simulink model "ThreePhasePFC_threePhase"  (R2018a)
settings: Solver=VariableStepAuto  StartTime=0.0  StopTime=0.6  RelTol=1e-3  AbsTol=1e-3  EnableMultiTasking=on
undefined symbols (not defined in the file or in its folder): Gain, L_Reactor, R_Reactor, Vac, Vdc, Vdc_offset
libraries: powerlib x36, powerlib_meascontrol x3
settings Model: Creator=snow_  LastModifiedBy=snow_
settings SolverCC: AutoScaleAbsTol=off
settings DataIOCC: LimitDataPoints=on  MaxDataPoints=10000
settings OptimizationCC: LifeSpan=inf
settings DebuggingCC: AllowSymbolicDim=off  SFUnexpectedBacktrackingDiag=warning  SFNoUnconditionalDefaultTransitionDiag=warning  SFExecutionAtInitializationDiag=none
settings CodeAppCC: StateflowObjectComments=on
settings GRTTargetCC: TargetLangStandard=C89/C90 (ANSI)  GeneratePreprocessorConditionals=Disable all
settings ConfigComp: CovMetricSettings=dw  CovHtmlReporting=on  CovSaveCumulativeToWorkspaceVar=on  CovSaveSingleToWorkspaceVar=on  CovExternalEMLEnable=off  CovSFcnEnable=off
settings SimscapeCC: SimscapeLogType=all  SimscapeLogDataHistory=10000

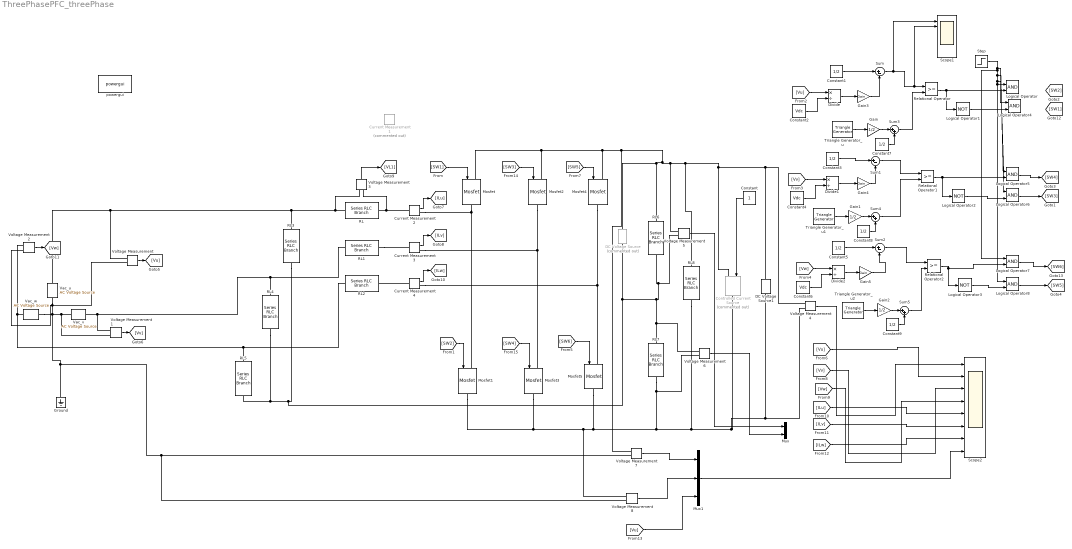
== system ThreePhasePFC_threePhase ==
  Constant : Constant
  Constant{1,3,5,7..9} (6 alike) : Constant  Value=1/2
  Constant2 : Constant  Value=Vdc
  Constant4 : Constant  Value=Vdc
  Constant6 : Constant  Value=Vdc
  Controlled Current Source : powerlib/Electrical Sources/Controlled Current Source  Commented=on  Initialize=on  Source_Type=AC  Amplitude=0  Phase=0  Frequency=0  Measurements=None
  Current Measurement1 : powerlib/Measurements/Current Measurement  Commented=on  PhasorSimulation=off  OutputType=Complex  PSBequivalent=0
  Current Measurement2 : powerlib/Measurements/Current Measurement  PhasorSimulation=off  OutputType=Complex  PSBequivalent=0
  Current Measurement3 : powerlib/Measurements/Current Measurement  PhasorSimulation=off  OutputType=Complex  PSBequivalent=0
  Current Measurement4 : powerlib/Measurements/Current Measurement  PhasorSimulation=off  OutputType=Complex  PSBequivalent=0
  DC Voltage Source : powerlib/Electrical Sources/DC Voltage Source  Commented=on  Amplitude=Vdc_offset  Measurements=None
  DC Voltage Source1 : powerlib/Electrical Sources/DC Voltage Source  Amplitude=Vdc  Measurements=None
  Divide : Product  Inputs=*/
  Divide1 : Product  Inputs=*/
  Divide2 : Product  Inputs=*/
  Gain : Gain  Gain=1/2
  Gain1 : Gain  Gain=1/2
  Gain2 : Gain  Gain=1/2
  Gain3 : Gain  Gain=Gain
  Gain4 : Gain  Gain=Gain
  Gain5 : Gain  Gain=Gain
  Ground : powerlib/Elements/Ground  LConnTagsString=a
  Logical Operator{,4..8} (6 alike) : Logic  AllPortsSameDT=off  OutDataTypeStr=boolean
  Logical Operator1 : Logic  Operator=NOT  AllPortsSameDT=off  OutDataTypeStr=boolean
  Logical Operator2 : Logic  Operator=NOT  AllPortsSameDT=off  OutDataTypeStr=boolean
  Logical Operator3 : Logic  Operator=NOT  AllPortsSameDT=off  OutDataTypeStr=boolean
  Mosfet{,1..5} (6 alike) : powerlib/Power Electronics/Mosfet  Ron=0.01  Lon=0  Rd=0.01  Vfd=0.7  IC=0  Rs=1e5  Cs=inf  Measurements=off
  Mux : Mux  Inputs=2
  Mux1 : Mux  Inputs=3
  RL : powerlib/Elements/Series RLC Branch  LConnTagsString=__new0  RConnTagsString=__new0  BranchType=RL  Resistance=R_Reactor  Inductance=L_Reactor  SetiL0=off  InitialCurrent=0  Capacitance=1e-6  Setx0=off  InitialVoltage=0  Measurements=None
      settings: AttributesFormatString=|
      | L=%<Inductance> H
      | R=%<Resistance> Ohm
  RL1 : powerlib/Elements/Series RLC Branch  LConnTagsString=__new0  RConnTagsString=__new0  BranchType=RL  Resistance=R_Reactor  Inductance=L_Reactor  SetiL0=off  InitialCurrent=0  Capacitance=1e-6  Setx0=off  InitialVoltage=0  Measurements=None
      settings: AttributesFormatString=|
      | L=%<Inductance> H
      | R=%<Resistance> Ohm
  RL2 : powerlib/Elements/Series RLC Branch  LConnTagsString=__new0  RConnTagsString=__new0  BranchType=RL  Resistance=R_Reactor  Inductance=L_Reactor  SetiL0=off  InitialCurrent=0  Capacitance=1e-6  Setx0=off  InitialVoltage=0  Measurements=None
      settings: AttributesFormatString=|
      | L=%<Inductance> H
      | R=%<Resistance> Ohm
  RL3 : powerlib/Elements/Series RLC Branch  LConnTagsString=__new0  RConnTagsString=__new0  BranchType=RC  Resistance=R_Reactor  Inductance=L_Reactor  SetiL0=off  InitialCurrent=0  Capacitance=20e-6  Setx0=off  InitialVoltage=0  Measurements=None
      settings: AttributesFormatString=C=%<Capacitance>F
  RL4 : powerlib/Elements/Series RLC Branch  LConnTagsString=__new0  RConnTagsString=__new0  BranchType=RC  Resistance=R_Reactor  Inductance=L_Reactor  SetiL0=off  InitialCurrent=0  Capacitance=20e-6  Setx0=off  InitialVoltage=0  Measurements=None
      settings: AttributesFormatString=C=%<Capacitance>F
  RL5 : powerlib/Elements/Series RLC Branch  LConnTagsString=__new0  RConnTagsString=__new0  BranchType=RC  Resistance=R_Reactor  Inductance=L_Reactor  SetiL0=off  InitialCurrent=0  Capacitance=20e-6  Setx0=off  InitialVoltage=0  Measurements=None
      settings: AttributesFormatString=C=%<Capacitance>F
  RL6 : powerlib/Elements/Series RLC Branch  LConnTagsString=__new0  RConnTagsString=__new0  BranchType=RC  Resistance=R_Reactor  Inductance=L_Reactor  SetiL0=off  InitialCurrent=0  Capacitance=20e-6  Setx0=on  InitialVoltage=Vdc/2  Measurements=None
      settings: AttributesFormatString=C=%<Capacitance>F
  RL7 : powerlib/Elements/Series RLC Branch  LConnTagsString=__new0  RConnTagsString=__new0  BranchType=RC  Resistance=R_Reactor  Inductance=L_Reactor  SetiL0=off  InitialCurrent=0  Capacitance=20e-6  Setx0=on  InitialVoltage=Vdc/2  Measurements=None
      settings: AttributesFormatString=C=%<Capacitance>F
  RL8 : powerlib/Elements/Series RLC Branch  LConnTagsString=__new0  RConnTagsString=__new0  BranchType=RC  Resistance=R_Reactor  Inductance=L_Reactor  SetiL0=off  InitialCurrent=0  Capacitance=1000e-6  Setx0=on  InitialVoltage=Vdc  Measurements=None
      settings: AttributesFormatString=C=%<Capacitance>F
  Relational Operator : RelationalOperator  OutDataTypeStr=boolean  RndMeth=Simplest
  Relational Operator1 : RelationalOperator  OutDataTypeStr=boolean  RndMeth=Simplest
  Relational Operator2 : RelationalOperator  OutDataTypeStr=boolean  RndMeth=Simplest
  Scope1 : Scope  NumInputPorts=8
  Scope2 : Scope  NumInputPorts=8
  Step : Step  Time=0.2  SampleTime=0
  Sum : Sum  Inputs=|+-
  Sum1 : Sum  Inputs=|+-
  Sum2 : Sum  Inputs=|+-
  Sum3 : Sum  Inputs=|++
  Sum4 : Sum  Inputs=|++
  Sum5 : Sum  Inputs=|++
  Triangle Generator_u : powerlib_meascontrol/Pulse & Signal Generators/Triangle Generator  Freq=60e3  Phase=0  Ts=0
  Triangle Generator_u1 : powerlib_meascontrol/Pulse & Signal Generators/Triangle Generator  Freq=60e3  Phase=-120  Ts=0
  Triangle Generator_u2 : powerlib_meascontrol/Pulse & Signal Generators/Triangle Generator  Freq=60e3  Phase=-240  Ts=0
  Vac_u : powerlib/Electrical Sources/AC Voltage Source  Amplitude=Vac*sqrt(2)  Phase=0  Frequency=50  SampleTime=0  Measurements=None  BusType=swing  Pref=10e3  Qref=0  Qmin=-inf  Qmax=+inf
      settings: AttributesFormatString=|
      | %<Amplitude> VoltPeak
      | %<Frequency> Hz
  Vac_v : powerlib/Electrical Sources/AC Voltage Source  Amplitude=Vac*sqrt(2)  Phase=-120  Frequency=50  SampleTime=0  Measurements=None  BusType=swing  Pref=10e3  Qref=0  Qmin=-inf  Qmax=+inf
      settings: AttributesFormatString=|
      | %<Amplitude> VoltPeak
      | %<Frequency> Hz
  Vac_w : powerlib/Electrical Sources/AC Voltage Source  Amplitude=Vac*sqrt(2)  Phase=-240  Frequency=50  SampleTime=0  Measurements=None  BusType=swing  Pref=10e3  Qref=0  Qmin=-inf  Qmax=+inf
      settings: AttributesFormatString=|
      | %<Amplitude> VoltPeak
      | %<Frequency> Hz
  Voltage Measurement{,1..8} (9 alike) : powerlib/Measurements/Voltage Measurement  PhasorSimulation=off  OutputType=Complex  PSBequivalent=0
  powergui : powerlib/powergui  Priority=1  SimulationMode=Continuous  SampleTime=50e-6  frequency=60  Iterations=50  frequencyindice=0  Pbase=100e6  ErrMax=1e-4  UnitsV=kV  UnitsW=MW  buscounter=0  FunctionMessages=off  echomessages=off  EnableUseOfTLC=off  CurrentSourceSwitches=off  DisableSnubberDevices=off  DisableRonSwitches=off  DisableVfSwitches=off  DisplayEquations=off  SolverType=Tustin/Backward Euler (TBE)  Interpol=off  ExternalGateDelay=off  methode=off  Ts=100  x0status=blocks  SPID=on  SwTol=0  HookPort=off  RestoreLinks=warning  ResistiveCurrentMeasurement=off  Frange=[0:2:500]  Ylog=off  Xlog=on  ShowGrid=off  save=off  variable=ZData  structure=0  ZoomFFT=off  StartTime=0.0  cycles=1  DisplayStyle=1  fundamental=60  FreqAxis=off  MaxFrequency=1000  frequencyindicesteady=1  RmsSteady=1  display=off
  wires:
  [SW2] -> Mosfet1/1
  Voltage Measurement/1 -> [Vu]
  Voltage Measurement3/1 -> [VL1]
  [SW1] -> Mosfet/1
  [SW3] -> Mosfet2/1
  [SW4] -> Mosfet3/1
  [SW6] -> Mosfet5/1
  [SW5] -> Mosfet4/1
  Current Measurement2/1 -> [ILu]
  Current Measurement3/1 -> [ILv]
  Current Measurement4/1 -> [ILw]
  Voltage Measurement1/1 -> [Vv]
  Voltage Measurement2/1 -> [Vw]
  Constant/1 -> Controlled Current Source/1
  [Vu] -> Divide/1
  Constant2/1 -> Divide/2
  Constant1/1 -> Sum/1
  Divide/1 -> Gain3/1
  Relational Operator/1 -> Logical Operator/2, Logical Operator1/1
  Sum/1 -> Scope1/1, Scope1/2, Relational Operator/1
  Constant4/1 -> Divide1/2
  Constant3/1 -> Sum1/1
  [Vv] -> Divide1/1
  Sum1/1 -> Relational Operator1/1
  Divide1/1 -> Gain4/1
  Divide2/1 -> Gain5/1
  Constant5/1 -> Sum2/1
  Sum2/1 -> Relational Operator2/1
  [Vw] -> Divide2/1
  Constant6/1 -> Divide2/2
  Relational Operator2/1 -> Logical Operator7/2, Logical Operator3/1
  Voltage Measurement4/1 -> Scope2/1
  [Vu] -> Scope2/2
  [Vv] -> Scope2/3
  [Vw] -> Scope2/4
  [ILu] -> Scope2/5
  [ILv] -> Scope2/6
  [ILw] -> Scope2/7
  Triangle Generator_u/1 -> Gain/1
  Constant7/1 -> Sum3/2
  Sum3/1 -> Relational Operator/2
  Gain/1 -> Sum3/1
  Triangle Generator_u1/1 -> Gain1/1
  Gain1/1 -> Sum4/1
  Constant8/1 -> Sum4/2
  Sum4/1 -> Relational Operator1/2
  Sum5/1 -> Relational Operator2/2
  Triangle Generator_u2/1 -> Gain2/1
  Gain2/1 -> Sum5/1
  Constant9/1 -> Sum5/2
  Voltage Measurement5/1 -> Mux/1
  Voltage Measurement6/1 -> Mux/2
  Logical Operator1/1 -> Logical Operator4/2
  Relational Operator1/1 -> Logical Operator5/2, Logical Operator2/1
  Logical Operator5/1 -> [SW4]
  Logical Operator2/1 -> Logical Operator6/2
  Logical Operator6/1 -> [SW3]
  Logical Operator7/1 -> [SW6]
  Logical Operator3/1 -> Logical Operator8/2
  Logical Operator8/1 -> [SW5]
  Step/1 -> Logical Operator6/1, Logical Operator7/1, Logical Operator8/1, Logical Operator/1, Logical Operator4/1, Logical Operator5/1
  Voltage Measurement7/1 -> Mux1/1
  Voltage Measurement8/1 -> Mux1/2
  [Vu] -> Mux1/3
  Mux1/1 -> Scope2/8
  Gain3/1 -> Sum/2
  Gain4/1 -> Sum1/2
  Gain5/1 -> Sum2/2
  connections:
  Mosfet1/RConn1 -- Voltage Measurement8/LConn1 -- Voltage Measurement6/LConn2 -- RL7/RConn1 -- DC Voltage Source1/LConn1 -- Voltage Measurement4/LConn2 -- Controlled Current Source/RConn1 -- RL8/RConn1 -- Mosfet5/RConn1 -- Mosfet3/RConn1
  Voltage Measurement3/LConn2 -- RL3/LConn1 -- Vac_u/RConn1 -- Voltage Measurement/LConn1 -- RL/LConn1
  Mosfet/RConn1 -- Current Measurement2/RConn1 -- Mosfet1/LConn1
  Mosfet2/LConn1 -- Mosfet/LConn1 -- Voltage Measurement7/LConn1 -- DC Voltage Source/RConn1 -- RL6/LConn1 -- Voltage Measurement5/LConn1 -- RL8/LConn1 -- DC Voltage Source1/RConn1 -- Voltage Measurement4/LConn1 -- Controlled Current Source/LConn1 -- Mosfet4/LConn1
  Mosfet4/RConn1 -- Current Measurement4/RConn1 -- Mosfet5/LConn1
  Mosfet2/RConn1 -- Current Measurement3/RConn1 -- Mosfet3/LConn1
  Vac_w/RConn1 -- Voltage Measurement2/LConn1 -- RL5/LConn1 -- RL2/LConn1
  Voltage Measurement3/LConn1 -- Current Measurement2/LConn1 -- RL/RConn1
  RL1/RConn1 -- Current Measurement3/LConn1
  Current Measurement4/LConn1 -- RL2/RConn1
  RL1/LConn1 -- Voltage Measurement1/LConn1 -- Vac_v/RConn1 -- RL4/LConn1
  RL7/LConn1 -- Voltage Measurement6/LConn1 -- DC Voltage Source/LConn1 -- RL4/RConn1 -- RL5/RConn1 -- RL3/RConn1 -- Voltage Measurement5/LConn2 -- RL6/RConn1
  Vac_v/LConn1 -- Voltage Measurement8/LConn2 -- Voltage Measurement7/LConn2 -- Ground/LConn1 -- Vac_u/LConn1 -- Voltage Measurement2/LConn2 -- Voltage Measurement/LConn2 -- Vac_w/LConn1 -- Voltage Measurement1/LConn2
